simulink model "DroneControl_Mod2_MixTakeoff"  (R2020a)
settings: Solver=VariableStepAuto  StartTime=0.0  StopTime=25  RelTol=1e-3
values from neighbouring files (symbols this model uses):
  b = 0.4    [Takeoff.m]
  body_rate_0 = [0;0;0]    [Takeoff.m]
  Boundaries = [B1;B2;B3]    [Takeoff.m]
  CMz_drone = 0-CMz    [Takeoff.m]
  CMz_tank = D_d2t + CMz    [Takeoff.m]
  Euler_0 = [0;0;0]    [Takeoff.m]
  g = [0;0;-9.8]    [Takeoff.m]
  I_Drone = [0.3933,0.3933,0.76]    [Takeoff.m]
  I_Tank = CalItank(m_tank,0.4,0.1,0.4,i)    [Takeoff.m]
  J = 0.00062    [Takeoff.m]
  K = 0.074    [Takeoff.m]
  k_T = MaxMotorThrsut/(MaxRPM^2)    (= 6.99167657551e-06)    [Takeoff.m]
  k_Thrsut2Torque = 0.021    [Takeoff.m]
  l = 0.5    [Takeoff.m]
  L = sqrt((x2-x1)^2 + (y2-y1)^2)    [Takeoff.m]
  m = m_drone + m_tank*percent    (= 36)    [Takeoff.m]    (also in animation.m = T_V1toI*T_V2toV1*T_BtoV2)
  m_drone = 20    [Takeoff.m]
  m_tank = 16    [Takeoff.m]
  MaxThrust = 4*MaxMotorThrsut    (= 529.2)    [Takeoff.m]
  MaxTilt = 30*pi/180    (= 0.523598775598)    [Takeoff.m]
  MaxTorque_XY = (T2-T1)*(l/sqrt(2))    [Takeoff.m]
  MaxVel = 1.5    [Takeoff.m]
  MaxVolt = 48    [Takeoff.m]
  MaxYawRate = 100*pi/180    (= 1.74532925199)    [Takeoff.m]
  MaxZVel = 2    [Takeoff.m]
  percent = 1    [Takeoff.m]
  R = 0.0062    [Takeoff.m]
  Target = WayPts(3,:)    [Takeoff.m]
  ts = 0.01    [Takeoff.m]
  WayPts = [[XYZ_0(1) XYZ_0(2) XYZ_0(3)] ... (first row only)    [Takeoff.m]
  XYZ_0 = [0;0;0]    [Takeoff.m]
undefined symbols (not defined in the file or in its folder): DiscIntNeverNeededParam, P1, P2, P3, P4, P5
libraries: simulink x23, vrlib x2, aerolibutil x1
(part 3 of 3)

== matlab function DroneControl_Mod2_MixTakeoff/Controller/MATLAB Function ==
  data: Xe input; xb output; Ye input; psi input; yb output
function [xb,yb] = fcn(Xe,Ye,psi)
    m = [[cos(psi) sin(psi)];[-sin(psi) cos(psi)]]
    pos = m*[Xe;Ye]
    xb = pos(1)
    yb = pos(2)

== matlab function DroneControl_Mod2_MixTakeoff/XYZsignal ==
  data: Xcmd input; RefXYZ output; Ycmd input; Zcmd input
function RefXYZ = fcn(Xcmd,Ycmd,Zcmd)

RefXYZ = [Xcmd;Ycmd;Zcmd]

== matlab function DroneControl_Mod2_MixTakeoff/6dof_system/ItoBTransform ==
  data: phi input; m output; theta input; psi input
function m = fcn(phi,theta,psi)
    T_ItoV1 = [[cos(psi) sin(psi) 0];[-sin(psi) cos(psi) 0];[0 0 1]]; 
    T_V1toV2 = [[cos(theta) 0 -sin(theta)];[0 1 0];[sin(theta) 0 cos(theta)]];
    T_V2toB = [[1 0 0];[0 cos(phi) sin(phi)];[0 -sin(phi) cos(phi)]];
    m = T_V2toB*T_V1toV2*T_ItoV1

== matlab function DroneControl_Mod2_MixTakeoff/WayPts to XYZerror ==
  data: waypts input; XYZerror output; XYZ input
function XYZerror = fcn(waypts,XYZ)
Xerror = waypts(1)-XYZ(1);
Yerror = waypts(2)-XYZ(2);
Zerror = waypts(3)-XYZ(3);
XYZerror = [Xerror;Yerror;Zerror];

== matlab function DroneControl_Mod2_MixTakeoff/Controller/ChangeMode ==
  data: XYZ input; Target input; SenseDist input; j input; mode input; action output; MaxVel input
function action = fcn(XYZ,Target,SenseDist,j,mode,MaxVel)
action = 0;
SafeZone = 1.0; % Fixed safezone based on the size of drone (drone size = 0.5)

% Approaching Mode
if mode == 0 && SenseDist < SafeZone + (0.85*MaxVel-0.075) % SafeZone + Deccleration Distance
   action = 1;
end

% Over Obstacle Mode
if mode == 1 && SenseDist > 0 + 0.7 && j < 0 % 0 is the basic trigger point
    action = 1;
end
if mode == 2 && SenseDist > 0 + 0.7 && j < 0
    action = 1;
end

% Leaving Mode
if mode == 3 && abs(Target(2)-XYZ(2)) < 0 + (0.85*MaxVel-0.075) 
    action = 1;
end

== matlab function DroneControl_Mod2_MixTakeoff/Controller/MATLAB Function1 ==
  data: Pos input; SensePt output; Bound input; SenseDist output; j output
function [SensePt,SenseDist,j] = fcn(Pos,Bound)
if length(Bound) > 1
    bx = Bound(1);
    by = Bound(2);
    tx = Bound(3);
    ty = Bound(4);
    nx = Bound(5);
    ny = Bound(6);
    X = Pos(1);
    Y = Pos(2);
    Z = Pos(3);

    j = ((ty*bx-tx*by)-(ty*X-tx*Y))/(ty*nx-tx*ny);
    SensePt = [X+nx*j;Y+ny*j;Z+0];
    SenseDist = sqrt((nx*j)^2 + (ny*j)^2);
else
    SensePt = [0;0;0];
    SenseDist = 999;
    j = 999;
end
